simulink model "inLoopSimu_pid"  (R2024a)
settings: Solver=FixedStepAuto  StartTime=0.0  StopTime=20000  FixedStep=1E-4  RelTol=1e-3
values from neighbouring files (symbols this model uses):
  initial_1 =     [ma.mat]    (also in regulation.mat)
  x = [input(1);input(2);input(3)]    [Dist_observer.m]    (also in is501nmtbModel_simu.m; is501nmtbModel_simu1.m; ma.mat = ; neuronalPID.m = entr(4))
  y = [input(7),input(8),input(9)]'    [estimator.m]    (also in is501nmtbModel_simu.m = B * x; is501nmtbModel_simu1.m = B * x + Td; ma.mat = ; regulation.mat = )
  z =     [ma.mat]    (also in regulation.mat)
undefined symbols (not defined in the file or in its folder): IAU
libraries: aerolibtransform2 x1, simulink x1
settings Model: Creator=b_ant  LastModifiedBy=b_ant

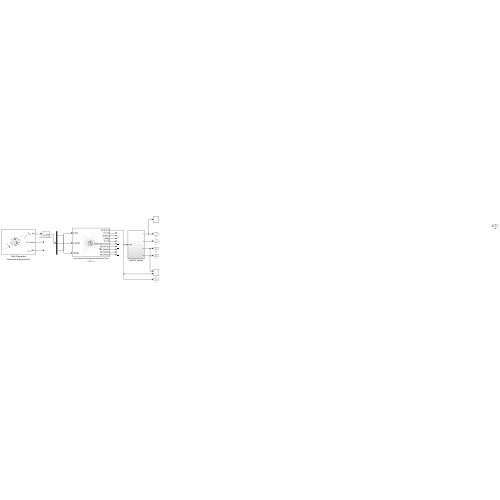
[thumbnail: Simulink's stored preview of the top-level diagram]
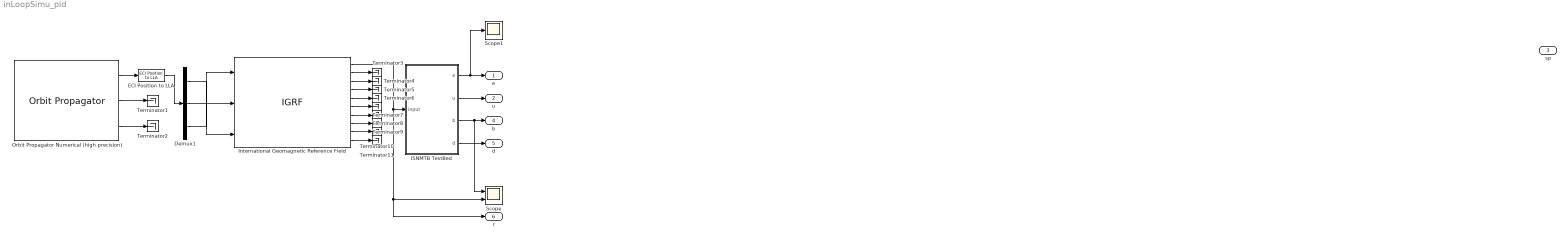
== system inLoopSimu_pid ==
  Demux1 : Demux  Outputs=3
  ECI Position to LLA : aerolibtransform2/ECI Position to LLA  red=IAU-2000/2006  year=2020  month=January  day=1  hour=0  min=0  sec=0  deltaT=None  errorflag=Error  extraparamflag=off  eunits=Metric (MKS)  earthmodel=WGS84  flat=1/298.257223563  eqradius=6378137
      settings: AttributesFormatString=%<red>
  ISNMTB TestBed : Subsystem
  International Geomagnetic Reference Field : IGRF  time_in=off  month=January  day=1  year=2020
      settings: AttributesFormatString=%<generation>
  Orbit Propagator Numerical (high precision) : OrbitPropagator  accelFrame=Fixed-frame  outportFrame=Fixed-frame  semiMajorAxis=orbit.semiMajorAxis  eccentricity=orbit.eccentricity  inclination=orbit.inclination  raan=orbit.rightAscensionOfAscendingNode  argPeriapsis=orbit.argumentOfPeriapsis  trueAnomaly=orbit.trueAnomaly  inertialPosition=[3649700.0 3308200.0 -4676600.0]  inertialVelocity=[-2750.8 6666.4 2573.4]  fixedPosition=[-4142689.0 -2676864.7 -4669861.6]  fixedVelocity=[1452.7 -6720.7 2568.1]  gravityModel=None  customR=3396200  customMu=4.305e13  customJ2=1.0826269e-03  customOmega=4.06125949e-3  outputTransform=on
  Scope : Scope  NumInputPorts=2
  Scope1 : Scope
  Terminator{1..11} (11 alike) : Terminator
  e : Outport
  u : Outport  Port=2
  sp : Outport  Port=3
  b : Outport  Port=4
  d : Outport  Port=5
  r : Outport  Port=6
  wires:
  Orbit Propagator Numerical (high precision)/3 -> Terminator2/1
  Orbit Propagator Numerical (high precision)/1 -> ECI Position to LLA/1
  Demux1/1 -> International Geomagnetic Reference Field/2
  Orbit Propagator Numerical (high precision)/2 -> Terminator1/1
  ECI Position to LLA/1 -> Demux1/1
  Demux1/3 -> International Geomagnetic Reference Field/1
  Demux1/2 -> International Geomagnetic Reference Field/3
  International Geomagnetic Reference Field/2 -> Terminator3/1
  International Geomagnetic Reference Field/3 -> Terminator4/1
  International Geomagnetic Reference Field/4 -> Terminator5/1
  International Geomagnetic Reference Field/5 -> Terminator6/1
  International Geomagnetic Reference Field/6 -> Terminator7/1
  International Geomagnetic Reference Field/7 -> Terminator8/1
  International Geomagnetic Reference Field/8 -> Terminator9/1
  International Geomagnetic Reference Field/9 -> Terminator10/1
  International Geomagnetic Reference Field/10 -> Terminator11/1
  International Geomagnetic Reference Field/1 -> r/1, Scope/2, ISNMTB TestBed/1(input)
  ISNMTB TestBed/1(e) -> Scope1/1, e/1
  ISNMTB TestBed/2(u) -> u/1
  ISNMTB TestBed/3(b) -> b/1, Scope/1
  ISNMTB TestBed/4(d) -> d/1

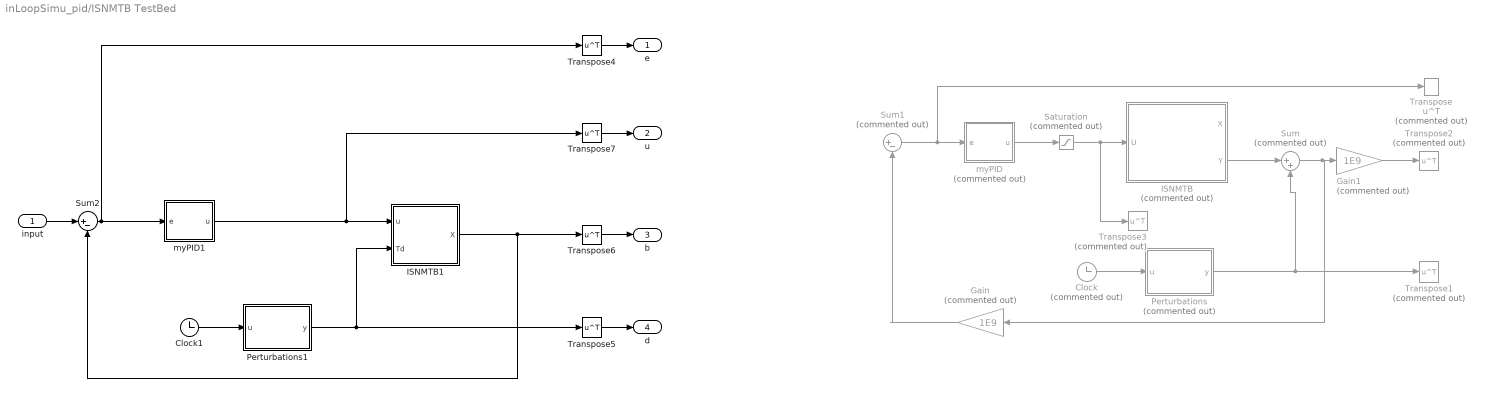
== system inLoopSimu_pid/ISNMTB TestBed ==
  input : Inport
  Clock : Clock  Commented=on
      settings: Decimation=1000
  Clock1 : Clock
      settings: Decimation=1000
  Gain : Gain  Commented=on  Gain=1E9
  Gain1 : Gain  Commented=on  Gain=1E9
  ISNMTB : Subsystem  Commented=on
  ISNMTB1 : Subsystem
  Perturbations : MATLAB Function  Commented=on  TreatAsAtomicUnit=on
  Perturbations1 : MATLAB Function  TreatAsAtomicUnit=on
  Saturation : Saturate  Commented=on  UpperLimit=[15,7,20]'  LowerLimit=[-15,-7,-25]'
  Sum : Sum  Commented=on  Inputs=|++
  Sum1 : Sum  Commented=on  Inputs=|+-
  Sum2 : Sum  Inputs=|+-
  Transpose{,1..3} (4 alike) : Math  Commented=on  Operator=transpose
  Transpose{4..7} (4 alike) : Math  Operator=transpose
  myPID : Subsystem  Commented=on
  myPID1 : Subsystem
  e : Outport
  u : Outport  Port=2
  b : Outport  Port=3
  d : Outport  Port=4
  wires:
  Sum1/1 -> Transpose/1, myPID/1(e)
  Gain/1 -> Sum1/2
  ISNMTB/2(Y) -> Sum/1
  Saturation/1 -> ISNMTB/1(U), Transpose3/1
  Clock/1 -> Perturbations/1(u)
  Gain1/1 -> Transpose2/1
  myPID/1(u) -> Saturation/1
  Perturbations/1(y) -> Sum/2, Transpose1/1
  Sum/1 -> Gain/1, Gain1/1
  Transpose6/1 -> b/1
  Transpose7/1 -> u/1
  Transpose4/1 -> e/1
  myPID1/1(u) -> Transpose7/1, ISNMTB1/1(u)
  Clock1/1 -> Perturbations1/1(u)
  Sum2/1 -> myPID1/1(e), Transpose4/1
  Perturbations1/1(y) -> Transpose5/1, ISNMTB1/2(Td)
  ISNMTB1/1(X) -> Transpose6/1, Sum2/2
  input/1 -> Sum2/1
  Transpose5/1 -> d/1

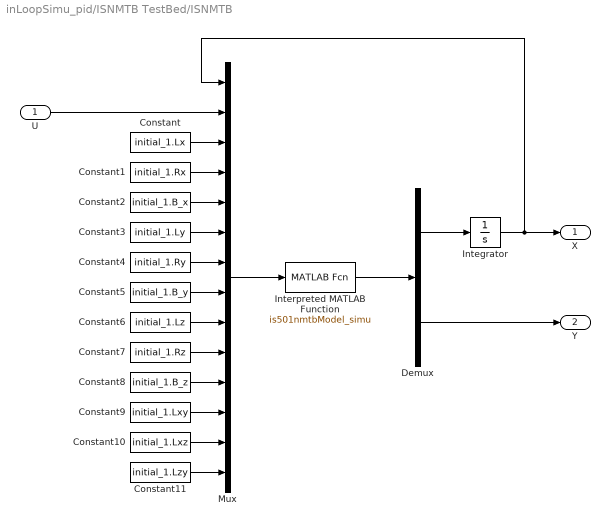
== system inLoopSimu_pid/ISNMTB TestBed/ISNMTB ==
  U : Inport
  Constant : Constant  Value=initial_1.Lx
  Constant1 : Constant  Value=initial_1.Rx
  Constant10 : Constant  Value=initial_1.Lxz
  Constant11 : Constant  Value=initial_1.Lzy
  Constant2 : Constant  Value=initial_1.B_x
  Constant3 : Constant  Value=initial_1.Ly
  Constant4 : Constant  Value=initial_1.Ry
  Constant5 : Constant  Value=initial_1.B_y
  Constant6 : Constant  Value=initial_1.Lz
  Constant7 : Constant  Value=initial_1.Rz
  Constant8 : Constant  Value=initial_1.B_z
  Constant9 : Constant  Value=initial_1.Lxy
  Demux : Demux  Outputs=2
  Integrator : Integrator  InitialCondition=[0,0,0]
  Interpreted MATLAB Function : MATLABFcn  MATLABFcn=is501nmtbModel_simu  OutputDimensions=6
  Mux : Mux  Inputs=14
  X : Outport
  Y : Outport  Port=2
  wires:
  Constant2/1 -> Mux/5
  Constant/1 -> Mux/3
  Demux/1 -> Integrator/1
  Interpreted MATLAB Function/1 -> Demux/1
  Constant9/1 -> Mux/12
  Constant5/1 -> Mux/8
  Constant3/1 -> Mux/6
  Constant1/1 -> Mux/4
  Integrator/1 -> X/1, Mux/1
  Mux/1 -> Interpreted MATLAB Function/1
  Constant10/1 -> Mux/13
  Constant7/1 -> Mux/10
  Constant11/1 -> Mux/14
  Constant4/1 -> Mux/7
  Constant8/1 -> Mux/11
  Constant6/1 -> Mux/9
  U/1 -> Mux/2
  Demux/2 -> Y/1

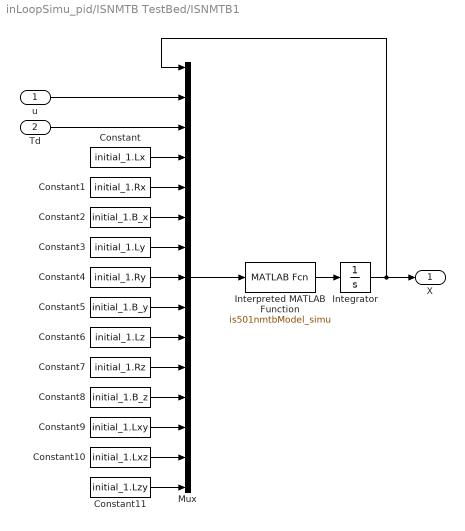
== system inLoopSimu_pid/ISNMTB TestBed/ISNMTB1 ==
  u : Inport
  Td : Inport  Port=2
  Constant : Constant  Value=initial_1.Lx
  Constant1 : Constant  Value=initial_1.Rx
  Constant10 : Constant  Value=initial_1.Lxz
  Constant11 : Constant  Value=initial_1.Lzy
  Constant2 : Constant  Value=initial_1.B_x
  Constant3 : Constant  Value=initial_1.Ly
  Constant4 : Constant  Value=initial_1.Ry
  Constant5 : Constant  Value=initial_1.B_y
  Constant6 : Constant  Value=initial_1.Lz
  Constant7 : Constant  Value=initial_1.Rz
  Constant8 : Constant  Value=initial_1.B_z
  Constant9 : Constant  Value=initial_1.Lxy
  Integrator : Integrator  InitialCondition=[3.249E4, -2.265E4, 3.655E4]
  Interpreted MATLAB Function : MATLABFcn  MATLABFcn=is501nmtbModel_simu
  Mux : Mux  Inputs=15
  X : Outport
  wires:
  Interpreted MATLAB Function/1 -> Integrator/1
  Integrator/1 -> X/1, Mux/1
  Mux/1 -> Interpreted MATLAB Function/1
  u/1 -> Mux/2
  Td/1 -> Mux/3
  Constant/1 -> Mux/4
  Constant1/1 -> Mux/5
  Constant2/1 -> Mux/6
  Constant3/1 -> Mux/7
  Constant4/1 -> Mux/8
  Constant5/1 -> Mux/9
  Constant6/1 -> Mux/10
  Constant7/1 -> Mux/11
  Constant8/1 -> Mux/12
  Constant9/1 -> Mux/13
  Constant10/1 -> Mux/14
  Constant11/1 -> Mux/15

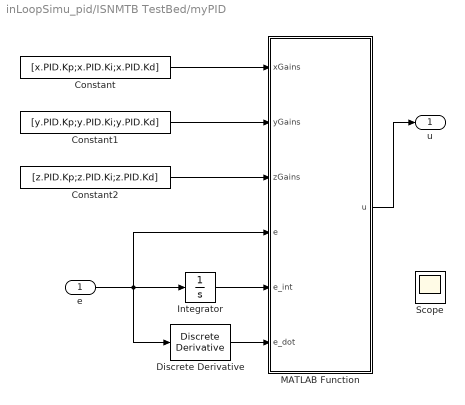
== system inLoopSimu_pid/ISNMTB TestBed/myPID ==
  e : Inport
  Constant : Constant  Value=[x.PID.Kp;x.PID.Ki;x.PID.Kd]
  Constant1 : Constant  Value=[y.PID.Kp;y.PID.Ki;y.PID.Kd]
  Constant2 : Constant  Value=[z.PID.Kp;z.PID.Ki;z.PID.Kd]
  Discrete Derivative : simulink/Discrete/Discrete Derivative  gainval=1.0  ICPrevScaledInput=0.0  OutMin=[]  OutMax=[]  OutDataType=fixdt(1, 16)  OutScaling=2^-10  DoSatur=off
  Integrator : Integrator
  MATLAB Function : MATLAB Function  TreatAsAtomicUnit=on
  Scope : Scope
  u : Outport
  wires:
  MATLAB Function/1(u) -> u/1
  e/1 -> Discrete Derivative/1, MATLAB Function/4(e), Integrator/1
  Discrete Derivative/1 -> MATLAB Function/6(e_dot)
  Integrator/1 -> MATLAB Function/5(e_int)
  Constant1/1 -> MATLAB Function/2(yGains)
  Constant/1 -> MATLAB Function/1(xGains)
  Constant2/1 -> MATLAB Function/3(zGains)
  ? -> Scope/1

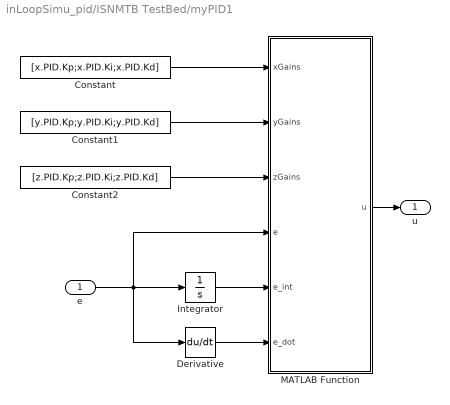
== system inLoopSimu_pid/ISNMTB TestBed/myPID1 ==
  e : Inport
  Constant : Constant  Value=[x.PID.Kp;x.PID.Ki;x.PID.Kd]
  Constant1 : Constant  Value=[y.PID.Kp;y.PID.Ki;y.PID.Kd]
  Constant2 : Constant  Value=[z.PID.Kp;z.PID.Ki;z.PID.Kd]
  Derivative : Derivative
  Integrator : Integrator
  MATLAB Function : MATLAB Function  TreatAsAtomicUnit=on
  u : Outport
  wires:
  MATLAB Function/1(u) -> u/1
  e/1 -> Derivative/1, MATLAB Function/4(e), Integrator/1
  Derivative/1 -> MATLAB Function/6(e_dot)
  Integrator/1 -> MATLAB Function/5(e_int)
  Constant1/1 -> MATLAB Function/2(yGains)
  Constant/1 -> MATLAB Function/1(xGains)
  Constant2/1 -> MATLAB Function/3(zGains)

== matlab function inLoopSimu_pid/ISNMTB TestBed/Perturbations1 ==
  data: u input; y output
function y = fcn(u)
y= [2.522*sin(2*pi*4.788E-3*u)+3.249E04;
   -5.174*sin(2*pi*7.481E-3*u)-2.265E04;
    3.359*sin(2*pi*8.378E-3*u)+3.655E04];
end

== matlab function inLoopSimu_pid/ISNMTB TestBed/Perturbations ==
  data: u input; y output
function y = fcn(u)
y= [2.522*sin(2*pi*4.788E-3*u)+3.249E04;
   -5.174*sin(2*pi*7.481E-3*u)-2.265E04;
    3.359*sin(2*pi*8.378E-3*u)+3.655E04]*1E-9;
end

== matlab function inLoopSimu_pid/ISNMTB TestBed/myPID1/MATLAB Function ==
  data: xGains input; u output; yGains input; zGains input; e input; e_int input; e_dot input
function u  = Bpid_controller(xGains, yGains, zGains, e, e_int, e_dot) 
    
    kp = diag([xGains(1),yGains(1),zGains(1)]);
    ki = diag([xGains(2),yGains(2),zGains(2)]);
    kd = diag([xGains(3),yGains(3),zGains(3)]);

    u=kp*e+ki*e_int+kd*e_dot;

end

== matlab function inLoopSimu_pid/ISNMTB TestBed/myPID/MATLAB Function ==
  data: xGains input; u output; yGains input; zGains input; e input; e_int input; e_dot input
function u  = Bpid_controller(xGains, yGains, zGains, e, e_int, e_dot) 
    
    kp = diag([xGains(1),yGains(1),zGains(1)]);
    ki = diag([xGains(2),yGains(2),zGains(2)]);
    kd = diag([xGains(3),yGains(3),zGains(3)]);

    u=kp*e+ki*e_int+kd*e_dot;

end
